simulink model "flyback"  (Simulink 6.1)
settings: Solver=ode23tb  StartTime=0.0  StopTime=0.001  MaxStep=1e-6  RelTol=1e-3  AbsTol=.01
libraries: powerlib x8
settings Model: LastModifiedBy=ThinkPad
settings DebuggingCC: SolverPrmCheckMsg=warning

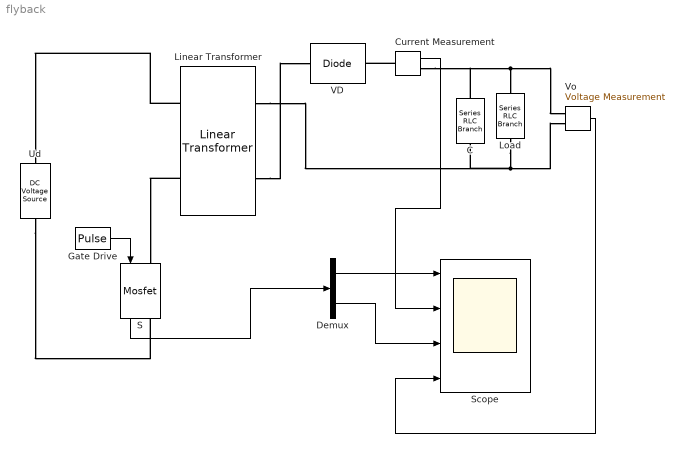
== system flyback ==
  C : powerlib/Elements/Series RLC Branch  Orientation=up  PhysicalDomain=powersysdomain  SubClassName=unknown  LeftPortType=p1  RightPortType=p1  LConnTagsString=__new0  RConnTagsString=__new0  Resistance=0  Inductance=0  Capacitance=1e-5  Measurements=None
  Current Measurement : powerlib/Measurements/Current Measurement  PhasorSimulation=off  OutputType=Complex  PSBequivalent=0
  Demux : Demux  Outputs=2
  Gate Drive : DiscretePulseGenerator  PulseType=Time based  Period=0.00005  PulseWidth=30
  Linear Transformer : powerlib/Elements/Linear Transformer  PhysicalDomain=powersysdomain  SubClassName=unknown  LeftPortType=p1  RightPortType=p1  LConnTagsString=a|b  RConnTagsString=A|B  NominalPower=[500 20e3 ]  winding1="[ 100  0.002  0.00001 ]"  winding2="[ 100  0.002  0.00001 ]"  ThreeWindings=off  winding3=[ 100 0.005 0.001 ]  RmLm=[ 100 1]  Measurements=Magnetization current
  Load : powerlib/Elements/Series RLC Branch  Orientation=down  PhysicalDomain=powersysdomain  SubClassName=unknown  LeftPortType=p1  RightPortType=p1  LConnTagsString=__new0  RConnTagsString=__new0  Resistance=100  Inductance=0  Capacitance=inf  Measurements=Branch voltage
  S : powerlib/Power Electronics/Mosfet  Orientation=down  Ron=0.01  Lon=1e-9  Rd=.01  IC=0  Rs=30  Cs=1e-9  Measurements=on
  Scope : Scope  NumInputPorts=4
      settings: TimeRange=0.0005  YMin=0~0~0~0  YMax=20~20~300~200  SampleTime=2e-4
  Ud : powerlib/Electrical Sources/DC Voltage Source  Orientation=up  Amplitude=100  Measurements=None
  VD : powerlib/Power Electronics/Diode  Ron=0.001  Lon=0  Vf=0  IC=0  Rs=100  Cs=1e-9  Measurements=off
  "Vo " : powerlib/Measurements/Voltage Measurement  PhasorSimulation=off  OutputType=Complex  PSBequivalent=0
  wires:
  Gate Drive/1 -> S/1
  S/1 -> Demux/1
  Demux/1 -> Scope/1
  Demux/2 -> Scope/3
  Current Measurement/1 -> Scope/2
  "Vo "/1 -> Scope/4
  connections:
  Ud/LConn1 -- S/RConn1
  Linear Transformer/LConn2 -- S/LConn1
  Linear Transformer/LConn1 -- Ud/RConn1
  Linear Transformer/RConn1 -- C/LConn1 -- "Vo "/LConn2 -- Load/RConn1
  Current Measurement/RConn1 -- C/RConn1 -- Load/LConn1 -- "Vo "/LConn1
  Linear Transformer/RConn2 -- VD/LConn1
  Current Measurement/LConn1 -- VD/RConn1
